simulink model "Sea_AdmittanceControl"  (R2025a)
settings: Solver=VariableStepAuto  StartTime=0.0  StopTime=50  RelTol=1e-3
undefined symbols (not defined in the file): bd, D, I, J, Jd, Jmotor, kd, ksea
libraries: slpidlib x1
settings Model: Creator=oskar  LastModifiedBy=oskar

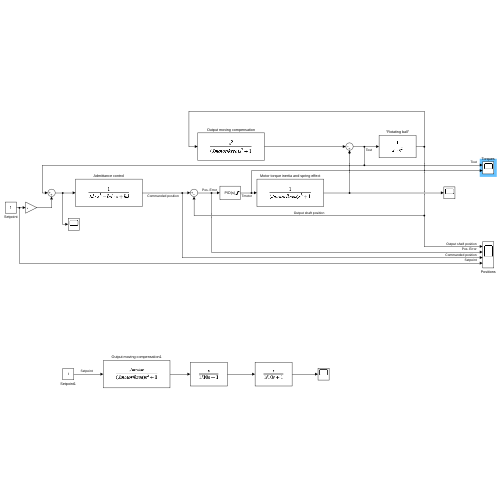
[thumbnail: Simulink's stored preview of the top-level diagram]
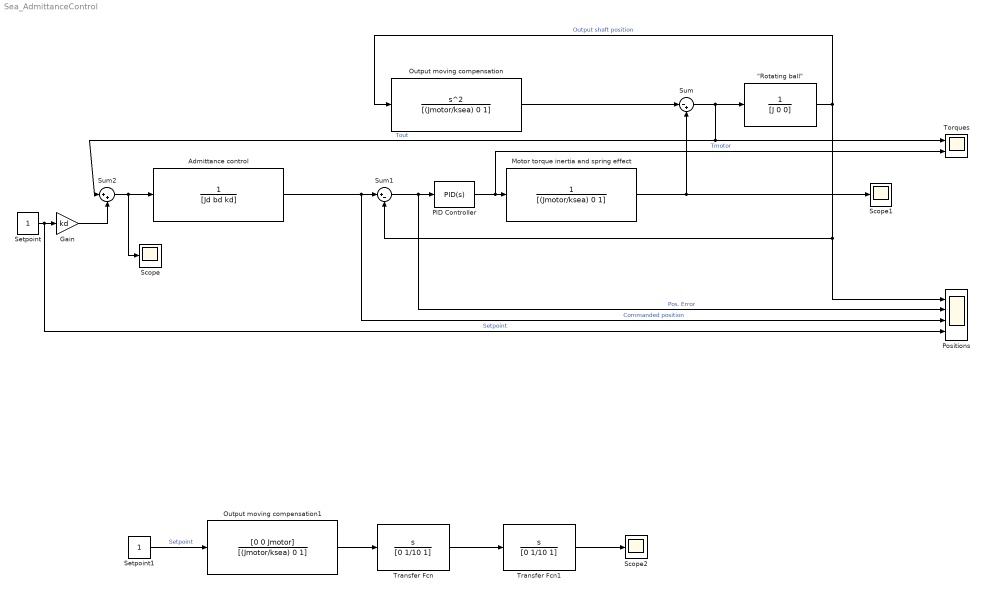
== system Sea_AdmittanceControl ==
  "\"Rotating ball\"" : TransferFcn  Numerator=[0 0 1]  Denominator=[J 0 0]
  Admittance control : TransferFcn  Denominator=[Jd bd kd]
  Gain : Gain  Gain=kd
  Motor torque inertia and spring effect : TransferFcn  Numerator=[0 0 1]  Denominator=[(Jmotor/ksea) 0 1]
  Output moving compensation : TransferFcn  Numerator=[1 0 0]  Denominator=[(Jmotor/ksea) 0 1]
  Output moving compensation1 : TransferFcn  Numerator=[0 0 Jmotor]  Denominator=[(Jmotor/ksea) 0 1]
  PID Controller : slpidlib/PID Controller  Controller=PID  Form=Parallel  TimeDomain=Continuous-time  UseExternalTs=off  SampleTime=-1  IntegratorMethod=Forward Euler  FilterMethod=Forward Euler  ControllerParametersSource=internal  P=1000  I=I  UseKiTs=off  D=D  UseExternalDerivativeSource=off  N=100  UseFilter=on  TunerSelectOption=Transfer Function Based (PID Tuner App)  InitialConditionSource=internal  InitialConditionForIntegrator=0  InitialConditionForFilter=0  DifferentiatorICPrevScaledInput=0  ExternalReset=none  TrackingMode=off  Kt=1  LimitOutput=on  SatLimitsSource=internal  UpperSaturationLimit=2  LowerSaturationLimit=-2  LinearizeAsGain=on  AntiWindupMode=none  Kb=1  LimitIntegrator=off  UpperIntegratorSaturationLimit=inf  LowerIntegratorSaturationLimit=-inf  POutMin=[]  POutMax=[]  IOutMin=[]  IOutMax=[]  DOutMin=[]  DOutMax=[]  NOutMin=[]  NOutMax=[]  SumOutMin=[]  SumOutMax=[]  SaturationOutMin=[]  SaturationOutMax=[]  PParamMin=[]  PParamMax=[]  IParamMin=[]  IParamMax=[]  DParamMin=[]  DParamMax=[]  NParamMin=[]  NParamMax=[]  KbParamMin=[]  KbParamMax=[]  KtParamMin=[]  KtParamMax=[]  KbOutMin=[]  KbOutMax=[]  KtOutMin=[]  KtOutMax=[]  IntegratorOutMin=[]  IntegratorOutMax=[]  FilterOutMin=[]  FilterOutMax=[]  SumI1OutMin=[]  SumI1OutMax=[]  SumI2OutMin=[]  SumI2OutMax=[]  SumI3OutMin=[]  SumI3OutMax=[]  SumI4OutMin=[]  SumI4OutMax=[]  SumDOutMin=[]  SumDOutMax=[]  DifferentiatorOutMin=[]  DifferentiatorOutMax=[]  FilterDiffOutCoefMin=[]  FilterDiffOutCoefMax=[]  ReciprocalOutMin=[]  ReciprocalOutMax=[]  SumDenOutMin=[]  SumDenOutMax=[]  SumNumOutMin=[]  SumNumOutMax=[]  DivideOutMin=[]  DivideOutMax=[]  UdiffTsProdOutMin=[]  UdiffTsProdOutMax=[]  NTsProdOutMin=[]  NTsProdOutMax=[]  UintegralTsProdOutMin=[]  UintegralTsProdOutMax=[]  UngainTsProdOutMin=[]  UngainTsProdOutMax=[]  ClampingZeroOutDataTypeStr=Inherit: Inherit via back propagation  ClampingZeroOutMin=[]  ClampingZeroOutMax=[]  FilterDenConstantOutDataTypeStr=Inherit: Inherit via back propagation  FilterDenConstantOutMin=[]  FilterDenConstantOutMax=[]  PCopyOutDataTypeStr=Inherit: Inherit via back propagation  PCopyOutMin=[]  PCopyOutMax=[]  NCopyOutDataTypeStr=Inherit: Inherit via back propagation  NCopyOutMin=[]  NCopyOutMax=[]  IntegratorContinuousStateAttributes=''  IntegratorStateMustResolveToSignalObject=off  IntegratorRTWStateStorageClass=Auto  FilterContinuousStateAttributes=''  FilterStateMustResolveToSignalObject=off  FilterRTWStateStorageClass=Auto  ParallelPVariant=InternalParameters  IdealPVariant=Disabled  IVariant=InternalParameters  DVariant=InternalParameters  IntegratorVariant=Continuous  SatVariant=Enabled  AWVariant=Passthrough  PCopyVariant=Disabled  TRVariant=Disabled  FdbkBlocksVariant=Forward  IdealPFdbkVariant=Disabled  SatFdbkVariant=Disabled  DerivativeFilterVariant=ContFilter  NVariant=InternalParameters  NCopyVariant=Disabled  FilterICVariant=InternalICsFilter  IntegratorICVariant=InternalICs  ExternalResetVariant=Disabled  TRSumVariant=Passthrough  SumFdbkVariant=Disabled  SumVariant=Sum_PID  TsampFilterVariant=InternalTs  TsampNgainVariant=Passthrough  TsampIntegralVariant=Disabled_SignalSpec  ExternalSaturationOutDataTypeStr=Inherit: Same as second input  DerivativeSourceVariant=ErrorSignal  PreIntVariant=InternalPreInt
  Positions : Scope  NumInputPorts=4
      settings: ActiveDisplayYMinimum=-2.5033046451582726  ActiveDisplayYMaximum=4.3699718469207607
  Scope : Scope
      settings: ActiveDisplayYMinimum=-453.57004481681838  ActiveDisplayYMaximum=1527.3201487105282  DataLoggingVariableName=ScopeData2
  Scope1 : Scope
      settings: ActiveDisplayYMinimum=-1  ActiveDisplayYMaximum=1  DataLoggingVariableName=ScopeData3
  Scope2 : Scope
      settings: ActiveDisplayYMinimum=-0.001671910435323162  ActiveDisplayYMaximum=0.00220002340894837  DataLoggingVariableName=ScopeData4
  Setpoint : Constant
  Setpoint1 : Constant
  Sum : Sum  Inputs=|-+
  Sum1 : Sum  Inputs=|+-
  Sum2 : Sum  Inputs=|++
  Torques : Scope  NumInputPorts=2
      settings: ActiveDisplayYMinimum=-5982.5543042774352  ActiveDisplayYMaximum=5979.4581019379248
  Transfer Fcn : TransferFcn  Numerator=[0 1 0]  Denominator=[0 1/10 1]
  Transfer Fcn1 : TransferFcn  Numerator=[0 1 0]  Denominator=[0 1/10 1]
  wires:
  Output moving compensation/1 -> Sum/1
  Motor torque inertia and spring effect/1 -> Scope1/1, Sum/2
  Sum/1 -> Torques/1, Sum2/1, "\"Rotating ball\""/1  "Tout"
  "\"Rotating ball\""/1 -> Positions/1, Sum1/2, Output moving compensation/1  "Output shaft position"
  PID Controller/1 -> Torques/2, Motor torque inertia and spring effect/1  "Tmotor"
  Sum1/1 -> Positions/2, PID Controller/1  "Pos. Error"
  Admittance control/1 -> Positions/3, Sum1/1  "Commanded position"
  Sum2/1 -> Admittance control/1, Scope/1
  Gain/1 -> Sum2/2
  Setpoint/1 -> Positions/4, Gain/1  "Setpoint"
  Setpoint1/1 -> Output moving compensation1/1  "Setpoint"
  Output moving compensation1/1 -> Transfer Fcn/1
  Transfer Fcn/1 -> Transfer Fcn1/1
  Transfer Fcn1/1 -> Scope2/1
